simulink model "init"  (R2019a)
settings: Solver=FixedStepAuto  StartTime=0.0  StopTime=10.0  FixedStep=1e-3  RelTol=1e-3
values from neighbouring files (symbols this model uses):
  den1 = [8 115 13]    [sys_ident.m]
  num1 = [11.25]    [sys_ident.m]
settings Model: Creator=DELL  LastModifiedBy=DELL

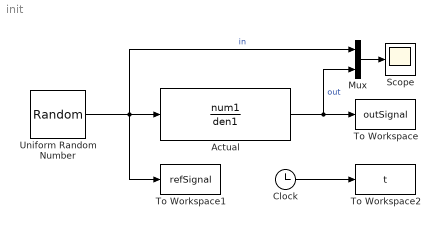
== system init ==
  Actual : TransferFcn  Numerator=num1  Denominator=den1
  Clock : Clock
  Mux : Mux  Inputs=2
  Scope : Scope
  To Workspace : ToWorkspace  VariableName=outSignal  SampleTime=-1
      settings: Save2DSignal=2-D array (concatenate along first dimension)
  To Workspace1 : ToWorkspace  VariableName=refSignal  SampleTime=-1
      settings: Save2DSignal=2-D array (concatenate along first dimension)
  To Workspace2 : ToWorkspace  VariableName=t  SampleTime=-1
      settings: Save2DSignal=2-D array (concatenate along first dimension)
  Uniform Random Number : UniformRandomNumber  SampleTime=1e-3  VectorParams1D=off
  wires:
  Uniform Random Number/1 -> To Workspace1/1, Mux/1, Actual/1  "in"
  Actual/1 -> To Workspace/1, Mux/2  "out"
  Mux/1 -> Scope/1
  Clock/1 -> To Workspace2/1
